simulink model "lr4"  (R2024a)
settings: Solver=ode23tb  StartTime=0.0  StopTime=1  MaxStep=1e-4  RelTol=1e-5
undefined symbols (not defined in the file): Control_Voltage, f_preobr, nagruzka
libraries: spsFourierLib x4, spsGroundLib x3, spsCurrentMeasurementLib x2, spsDCVoltageSourceLib x2, spsMultimeterLib x1, spsRMSLib x1, spsSeriesRLCBranchLib x1, simulink x1, spsUniversalBridgeLib x1, spsVoltageMeasurementLib x1, sps_lib x1
settings Model: Creator=79532  LastModifiedBy=79532

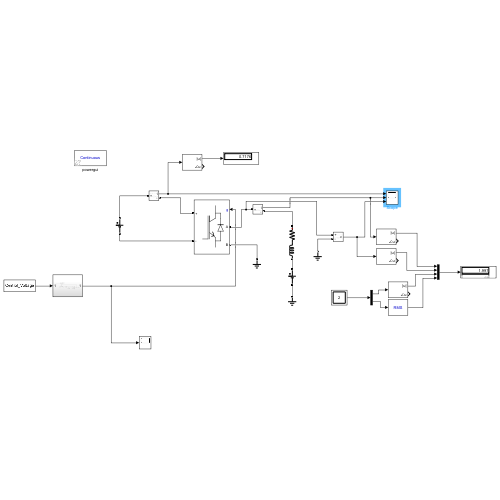
[thumbnail: Simulink's stored preview of the top-level diagram]
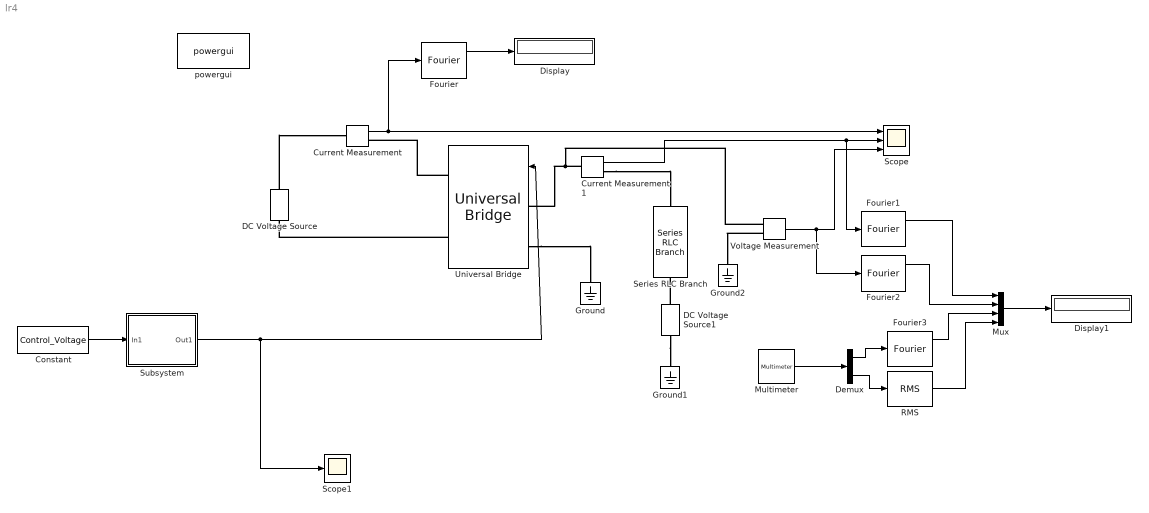
== system lr4 ==
  Constant : Constant  Value=Control_Voltage
  Current Measurement : spsCurrentMeasurementLib/Current Measurement  PhasorSimulation=off  OutputType=Complex  PSBequivalent=0
  Current Measurement1 : spsCurrentMeasurementLib/Current Measurement  PhasorSimulation=off  OutputType=Complex  PSBequivalent=0
  DC Voltage Source : spsDCVoltageSourceLib/DC Voltage Source  Amplitude=100  Measurements=None
  DC Voltage Source1 : spsDCVoltageSourceLib/DC Voltage Source  Amplitude=50  Measurements=None
  Demux : Demux  Outputs=2
  Display : Display
  Display1 : Display
  Fourier{,1..3} (4 alike) : spsFourierLib/Fourier  Freq=f_preobr  n=0  InInit=[0, 0]  Ts=0
  Ground : spsGroundLib/Ground  LConnTagsString=a
  Ground1 : spsGroundLib/Ground  LConnTagsString=a
  Ground2 : spsGroundLib/Ground  LConnTagsString=a
  Multimeter : spsMultimeterLib/Multimeter  L=10  sel=[1 7]  yselected={}  Gain=[1 1]  OutputType=Complex  PlotAtSimulationStop=off  PhasorSimulation=off
  Mux : Mux
  RMS : spsRMSLib/RMS  TrueRMS=on  Freq=f_preobr  RMSInit=0  Ts=0
  Scope : Scope  NumInputPorts=3
  Scope1 : Scope
  Series RLC Branch : spsSeriesRLCBranchLib/Series RLC Branch  LConnTagsString=__new0  RConnTagsString=__new0  BranchType=RL  Resistance=nagruzka.Res  Inductance=nagruzka.Ind  SetiL0=off  InitialCurrent=0  Capacitance=1e-6  Setx0=off  InitialVoltage=0  Measurements=None
  Subsystem : Subsystem
  Universal Bridge : spsUniversalBridgeLib/Universal Bridge  Arms=2  SnubberResistance=1e5  SnubberCapacitance=inf  Device=IGBT / Diodes  Ron=1e-3  Lon=0  ForwardVoltages="[  2  2  ]"  ForwardVoltage=0  GTOparameters=[ 10e-6 , 20e-6 ]  IGBTparameters=[ 1e-6 , 2e-6 ]  Measurements=All voltages and currents  Measurements_2=None  converterType=Rectifier
  Voltage Measurement : spsVoltageMeasurementLib/Voltage Measurement  PhasorSimulation=off  OutputType=Complex  PSBequivalent=0
  powergui : sps_lib/powergui  Priority=1  SimulationMode=Continuous  SampleTime=50e-6  frequency=60  Iterations=50  frequencyindice=0  Pbase=100e6  ErrMax=1e-4  UnitsV=kV  UnitsW=MW  buscounter=0  FunctionMessages=off  echomessages=off  EnableUseOfTLC=off  CurrentSourceSwitches=off  DisableSnubberDevices=off  DisableRonSwitches=off  DisableVfSwitches=off  DisplayEquations=off  AutomaticDiscreteSolvers=off  SolverType=Tustin/Backward Euler (TBE)  Interpol=off  ExternalGateDelay=off  methode=off  Ts=100  x0status=blocks  SPID=on  SwTol=0  HookPort=off  NonlinearTolerance=1e-4  nMaxIteration=100  ContinueOnMaxIteration=off  RestoreLinks=warning  ResistiveCurrentMeasurement=off  Frange=[0:2:500]  Ylog=off  Xlog=on  ShowGrid=off  save=off  variable=ZData  structure=0  ZoomFFT=off  StartTime=0.0  cycles=1  DisplayStyle=1  fundamental=60  FreqAxis=off  MaxFrequency=1000  frequencyindicesteady=1  RmsSteady=1  display=off
  wires:
  Current Measurement/1 -> Fourier/1, Scope/1
  Fourier/1 -> Display/1
  Current Measurement1/1 -> Fourier1/1, Scope/2
  Voltage Measurement/1 -> Fourier2/1, Scope/3
  Mux/1 -> Display1/1
  Fourier1/1 -> Mux/1
  Fourier2/1 -> Mux/2
  Multimeter/1 -> Demux/1
  Demux/2 -> RMS/1
  RMS/1 -> Mux/4
  Demux/1 -> Fourier3/1
  Fourier3/1 -> Mux/3
  Constant/1 -> Subsystem/1(In1)
  Subsystem/1(Out1) -> Scope1/1, Universal Bridge/1
  connections:
  DC Voltage Source/RConn1 -- Current Measurement/LConn1
  Universal Bridge/RConn1 -- Current Measurement/RConn1
  Universal Bridge/RConn2 -- DC Voltage Source/LConn1
  Current Measurement1/LConn1 -- Voltage Measurement/LConn1 -- Universal Bridge/LConn1
  Universal Bridge/LConn2 -- Ground/LConn1
  Current Measurement1/RConn1 -- Series RLC Branch/LConn1
  DC Voltage Source1/RConn1 -- Series RLC Branch/RConn1
  DC Voltage Source1/LConn1 -- Ground1/LConn1
  Voltage Measurement/LConn2 -- Ground2/LConn1

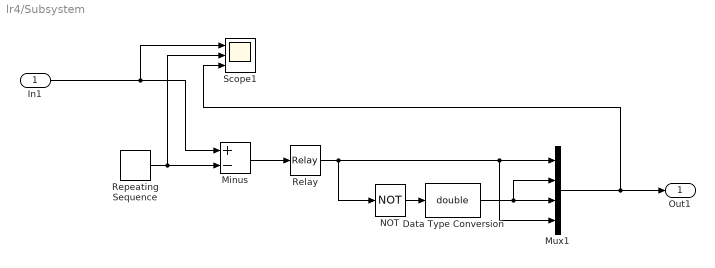
== system lr4/Subsystem ==
  In1 : Inport
  Data Type Conversion : DataTypeConversion  OutDataTypeStr=double  SaturateOnIntegerOverflow=off  RndMeth=Floor
  Minus : Sum  Inputs=+-
  Mux1 : Mux
  NOT : Logic  Operator=NOT  IconShape=distinctive  AllPortsSameDT=off  OutDataTypeStr=boolean
  Relay : Relay
  Repeating Sequence : simulink/Sources/Repeating Sequence  rep_seq_t=[0 0.5/f_preobr 1/f_preobr]  rep_seq_y=[-2 2 -2]
  Scope1 : Scope  NumInputPorts=3
  Out1 : Outport
  wires:
  Repeating Sequence/1 -> Scope1/2, Minus/2
  Relay/1 -> NOT/1, Mux1/4, Mux1/1
  Mux1/1 -> Scope1/3, Out1/1
  NOT/1 -> Data Type Conversion/1
  In1/1 -> Minus/1, Scope1/1
  Minus/1 -> Relay/1
  Data Type Conversion/1 -> Mux1/2, Mux1/3
